simulink model "Sim_Ex14"  (R2017a)
settings: Solver=VariableStepAuto  StartTime=0.0  StopTime=Stop_Time  MaxStep=1e-4  RelTol=1e-3
values from neighbouring files (symbols this model uses):
  Bm = 0    [A_Ex14.m]
  Jm = 0.001    [A_Ex14.m]
  Lamf = 0.254    [A_Ex14.m]
  Lds = 3.6e-3    (= 0.0036)    [A_Ex14.m]
  Lqs = 4.3e-3    (= 0.0043)    [A_Ex14.m]
  p = 3    [A_Ex14.m]
  Rs = 0.15    [A_Ex14.m]
  Thetarm_Init = 0*pi*1/p    (= 0)    [A_Ex14.m]
  Vdqsr = [0;Wr_Target*Lamf]    [A_Ex14.m]
  Wrm_Init = 0*2*pi/60    (= 0)    [A_Ex14.m]
settings Model: Creator=KYC  LastModifiedBy=KYC

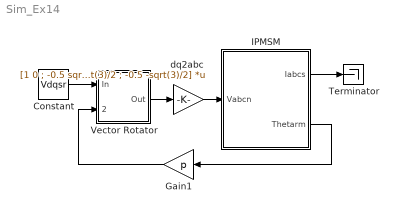
== system Sim_Ex14 ==
  Constant : Constant  Value=Vdqsr
  Gain1 : Gain  Gain=p
  IPMSM : Subsystem
  Terminator : Terminator
  Vector Rotator : Subsystem
  dq2abc : Gain  Gain=[1 0 ; -0.5 sqrt(3)/2 ; -0.5 -sqrt(3)/2]  Multiplication=Matrix(K*u)
  wires:
  Gain1/1 -> Vector Rotator/2(Theta)
  Constant/1 -> Vector Rotator/1(In)
  IPMSM/2(Thetarm) -> Gain1/1
  Vector Rotator/1(Out) -> dq2abc/1
  dq2abc/1 -> IPMSM/1(Vabcn)
  IPMSM/1(Iabcs) -> Terminator/1

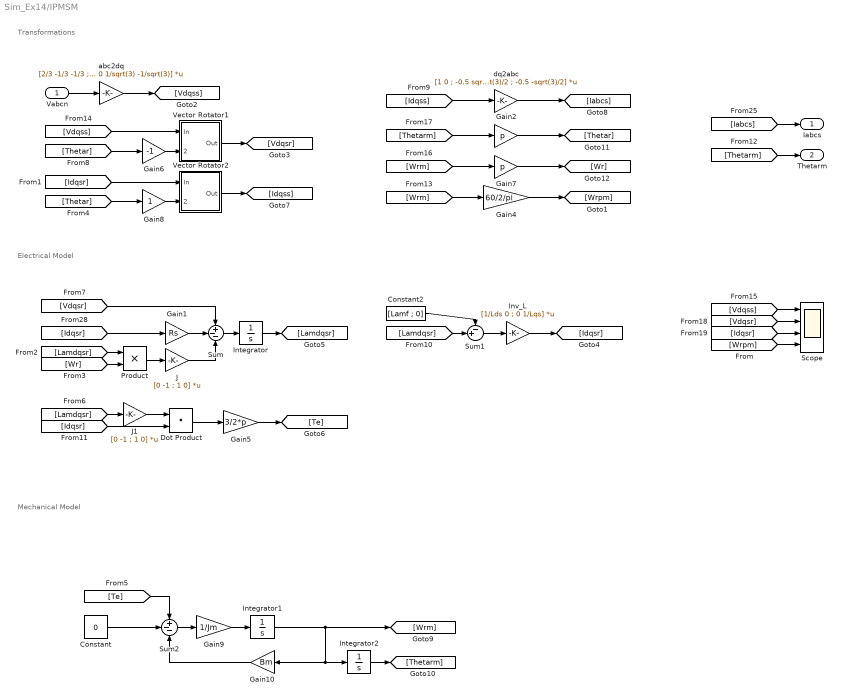
== system Sim_Ex14/IPMSM ==
  note: Transformations
  note: Electrical Model
  note: Mechanical Model
  Vabcn : Inport
  Constant : Constant  Value=0
  Constant2 : Constant  Value=[Lamf ; 0]
  Dot Product : DotProduct  InputSameDT=on  OutDataTypeStr=Inherit: Inherit via internal rule
  Gain1 : Gain  Gain=Rs
  Gain10 : Gain  Gain=Bm
  Gain2 : Gain  Gain=p
  Gain4 : Gain  Gain=60/2/pi
  Gain5 : Gain  Gain=3/2*p
  Gain6 : Gain  Gain=-1
  Gain7 : Gain  Gain=p
  Gain8 : Gain
  Gain9 : Gain  Gain=1/Jm
  Integrator : Integrator  InitialCondition=[Lamf ; 0]
  Integrator1 : Integrator  InitialCondition=Wrm_Init
  Integrator2 : Integrator  InitialCondition=Thetarm_Init  WrapState=on
  Inv_L : Gain  Gain=[1/Lds 0 ; 0 1/Lqs]  Multiplication=Matrix(K*u)
  J : Gain  Gain=[0 -1 ; 1 0]  Multiplication=Matrix(K*u)
  J1 : Gain  Gain=[0 -1 ; 1 0]  Multiplication=Matrix(K*u)
  Product : Product  RndMeth=Zero
  Scope : Scope  NumInputPorts=4
  Sum : Sum  Inputs=+--
  Sum1 : Sum  Inputs=-+|
  Sum2 : Sum  Inputs=+--
  Vector Rotator1 : Subsystem
  Vector Rotator2 : Subsystem
  abc2dq : Gain  Gain=[2/3 -1/3 -1/3 ; 0 1/sqrt(3) -1/sqrt(3)]  Multiplication=Matrix(K*u)  SaturateOnIntegerOverflow=on  OutDataTypeStr=Inherit: Same as input  ParamDataTypeStr=Inherit: Same as input
  dq2abc : Gain  Gain=[1 0 ; -0.5 sqrt(3)/2 ; -0.5 -sqrt(3)/2]  Multiplication=Matrix(K*u)
  Iabcs : Outport
  Thetarm : Outport  Port=2
  wires:
  [Iabcs] -> Iabcs/1
  [Wrm] -> Gain7/1
  [Thetarm] -> Gain2/1
  Gain7/1 -> [Wr]
  dq2abc/1 -> [Iabcs]
  [Idqss] -> dq2abc/1
  Vector Rotator2/1(Out) -> [Idqss]
  [Idqsr] -> Vector Rotator2/1(In)
  Vector Rotator1/1(Out) -> [Vdqsr]
  [Thetarm] -> Thetarm/1
  Gain2/1 -> [Thetar]
  [Thetar] -> Gain6/1
  Gain6/1 -> Vector Rotator1/2(Theta)
  [Thetar] -> Gain8/1
  Gain8/1 -> Vector Rotator2/2(Theta)
  Gain10/1 -> Sum2/3
  Integrator2/1 -> [Thetarm]
  [Te] -> Sum2/1
  Sum2/1 -> Gain9/1
  Constant/1 -> Sum2/2
  Integrator1/1 -> [Wrm], Integrator2/1, Gain10/1
  Gain9/1 -> Integrator1/1
  Sum1/1 -> Inv_L/1
  Inv_L/1 -> [Idqsr]
  [Lamdqsr] -> Sum1/2
  Constant2/1 -> Sum1/1
  Dot Product/1 -> Gain5/1
  J1/1 -> Dot Product/1
  [Lamdqsr] -> J1/1
  [Idqsr] -> Dot Product/2
  Gain5/1 -> [Te]
  Integrator/1 -> [Lamdqsr]
  [Vdqsr] -> Sum/1
  [Lamdqsr] -> Product/1
  Sum/1 -> Integrator/1
  [Wr] -> Product/2
  Product/1 -> J/1
  [Idqsr] -> Gain1/1
  J/1 -> Sum/3
  Gain1/1 -> Sum/2
  [Wrm] -> Gain4/1
  Gain4/1 -> [Wrpm]
  Vabcn/1 -> abc2dq/1
  [Vdqsr] -> Scope/2
  [Idqsr] -> Scope/3
  [Wrpm] -> Scope/4
  abc2dq/1 -> [Vdqss]
  [Vdqss] -> Vector Rotator1/1(In)
  [Vdqss] -> Scope/1

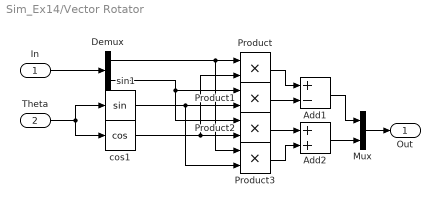
== system Sim_Ex14/Vector Rotator ==
  In : Inport
  Theta : Inport  Port=2
  Add1 : Sum  Inputs=+-
  Add2 : Sum
  Demux : Demux  Outputs=2
  Mux : Mux  Inputs=[1 1]
  Product{,1..3} (4 alike) : Product  RndMeth=Zero
  cos1 : Trigonometry  Operator=cos
  sin1 : Trigonometry
  Out : Outport
  wires:
  Add2/1 -> Mux/2
  Product3/1 -> Add2/2
  Product2/1 -> Add2/1
  Add1/1 -> Mux/1
  Product1/1 -> Add1/2
  Product/1 -> Add1/1
  sin1/1 -> Product3/2, Product1/2
  cos1/1 -> Product2/2, Product/2
  Demux/2 -> Product2/1, Product1/1
  In/1 -> Demux/1
  Mux/1 -> Out/1
  Demux/1 -> Product/1, Product3/1
  Theta/1 -> sin1/1, cos1/1

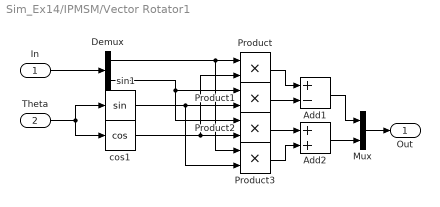
== system Sim_Ex14/IPMSM/Vector Rotator1 ==
  In : Inport
  Theta : Inport  Port=2
  Add1 : Sum  Inputs=+-
  Add2 : Sum
  Demux : Demux  Outputs=2
  Mux : Mux  Inputs=[1 1]
  Product{,1..3} (4 alike) : Product  RndMeth=Zero
  cos1 : Trigonometry  Operator=cos
  sin1 : Trigonometry
  Out : Outport
  wires:
  Add2/1 -> Mux/2
  Product3/1 -> Add2/2
  Product2/1 -> Add2/1
  Add1/1 -> Mux/1
  Product1/1 -> Add1/2
  Product/1 -> Add1/1
  sin1/1 -> Product3/2, Product1/2
  cos1/1 -> Product2/2, Product/2
  Demux/2 -> Product2/1, Product1/1
  In/1 -> Demux/1
  Mux/1 -> Out/1
  Demux/1 -> Product/1, Product3/1
  Theta/1 -> sin1/1, cos1/1

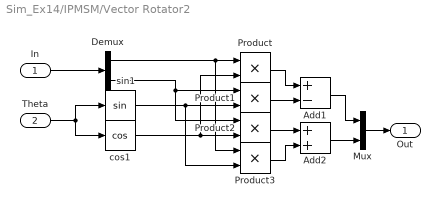
== system Sim_Ex14/IPMSM/Vector Rotator2 ==
  In : Inport
  Theta : Inport  Port=2
  Add1 : Sum  Inputs=+-
  Add2 : Sum
  Demux : Demux  Outputs=2
  Mux : Mux  Inputs=[1 1]
  Product{,1..3} (4 alike) : Product  RndMeth=Zero
  cos1 : Trigonometry  Operator=cos
  sin1 : Trigonometry
  Out : Outport
  wires:
  Theta/1 -> cos1/1, sin1/1
  Demux/1 -> Product3/1, Product/1
  Mux/1 -> Out/1
  In/1 -> Demux/1
  Demux/2 -> Product1/1, Product2/1
  cos1/1 -> Product/2, Product2/2
  sin1/1 -> Product1/2, Product3/2
  Product/1 -> Add1/1
  Product1/1 -> Add1/2
  Add1/1 -> Mux/1
  Product2/1 -> Add2/1
  Product3/1 -> Add2/2
  Add2/1 -> Mux/2
